simulink model "bic_2"  (R2018a)
settings: Solver=FixedStepAuto  StartTime=0.0  StopTime=10.0  FixedStep=Ts  RelTol=1e-3  EnableMultiTasking=on
values from neighbouring files (symbols this model uses):
  delta_f = alpha    [sim_veh_MPC.m]
  psi0 = psi    (= 3.14159265359)    [sim_veh_MPC.m]
  v_cmd = v    [sim_veh_MPC.m]
  x_car0 = x_car    (= 80)    [sim_veh_MPC.m]
  y_car0 = y_car    (= 30)    [sim_veh_MPC.m]
libraries: simulink x1
settings Model: Creator=Administrator  LastModifiedBy=berlin
settings DataIOCC: LimitDataPoints=on  SaveFormat=Array
settings OptimizationCC: LifeSpan=inf
settings DebuggingCC: SolverPrmCheckMsg=warning  SFUnexpectedBacktrackingDiag=warning  SFNoUnconditionalDefaultTransitionDiag=warning  SFExecutionAtInitializationDiag=none
settings HardwareCC: ProdBitPerPointer=32  ProdBitPerSizeT=32  ProdBitPerPtrDiffT=32  ProdLargestAtomicFloat=None  ProdIntDivRoundTo=Undefined  ProdEndianess=Unspecified  ProdWordSize=32  ProdHWDeviceType=32-bit Generic
settings ModelReferenceCC: PropagateSignalLabelsOutOfModel=off
settings CodeAppCC: StateflowObjectComments=on
settings GRTTargetCC: TargetLangStandard=C89/C90 (ANSI)  GeneratePreprocessorConditionals=Disable all
settings ConfigComp: CovMetricSettings=dw  CovHtmlReporting=on  CovSaveCumulativeToWorkspaceVar=on  CovSaveSingleToWorkspaceVar=on  CovExternalEMLEnable=off  CovSFcnEnable=off

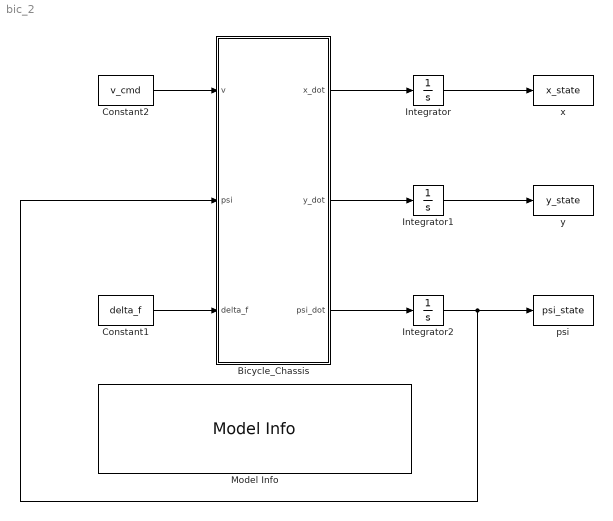
== system bic_2 ==
  " Bicycle_Chassis" : MATLAB Function  TreatAsAtomicUnit=on
  Constant1 : Constant  Value=delta_f
  Constant2 : Constant  Value=v_cmd
  Integrator : Integrator  InitialCondition=x_car0
  Integrator1 : Integrator  InitialCondition=y_car0
  Integrator2 : Integrator  InitialCondition=psi0
  Model Info : simulink/Model-Wide Utilities/Model Info  Frame=on  DisplayStringWithTags=|  HorizontalTextAlignment=Left  LeftAlignmentValue=0.02
      | Model Info
      | 
      | [delta_f] is the steering angle on the front wheels.
      | Closewise is Positive.
      | 
      | [acc] is the acceleration requirement.
  psi : ToWorkspace  VariableName=psi_state  SaveFormat=Timeseries  SampleTime=-1
  x : ToWorkspace  VariableName=x_state  SaveFormat=Timeseries  SampleTime=-1
  y : ToWorkspace  VariableName=y_state  SaveFormat=Timeseries  SampleTime=-1
  wires:
  " Bicycle_Chassis"/1(x_dot) -> Integrator/1
  " Bicycle_Chassis"/2(y_dot) -> Integrator1/1
  " Bicycle_Chassis"/3(psi_dot) -> Integrator2/1
  Integrator2/1 -> psi/1, " Bicycle_Chassis"/2(psi)
  Integrator/1 -> x/1
  Integrator1/1 -> y/1
  Constant1/1 -> " Bicycle_Chassis"/3(delta_f)
  Constant2/1 -> " Bicycle_Chassis"/1(v)

== matlab function bic_2/ Bicycle_Chassis ==
  data: v input; x_dot output; psi input; delta_f input; y_dot output; psi_dot output
function [x_dot,y_dot,psi_dot] = bicycle(v, psi,delta_f)

lr = 1.6;
lf = 1.4;
wb = lr+lf;
beta = atan(lr/wb*tan(delta_f));

x_dot = v*cos(psi+ beta);
y_dot = v*sin(psi+beta);
psi_dot= v/lr*sin(beta);

end

%% ref: http://www.me.berkeley.edu/~frborrel/pdfpub/IV_KinematicMPC_jason.pdf
